simulink model "Final_openloop"  (R2024b)
settings: Solver=ode23s  StartTime=0.0  StopTime=150  RelTol=1e-3
(part 1 of 2)
settings Model: Creator=thomasmacbookpro  LastModifiedBy=thomasmacbookpro
settings OptimizationCC: ReuseModelBlockBuffer=off
settings RTWCC: GPUComputeCapability=3.5

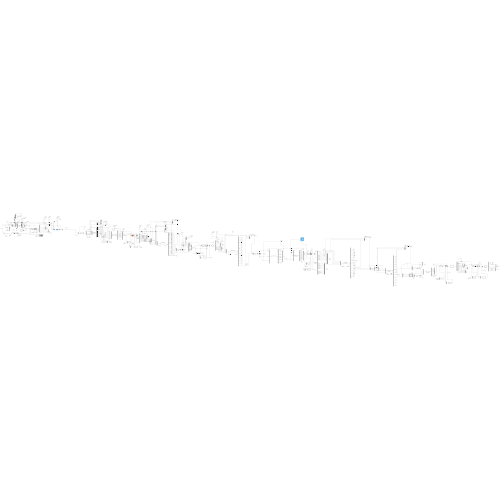
[thumbnail: Simulink's stored preview of the top-level diagram]
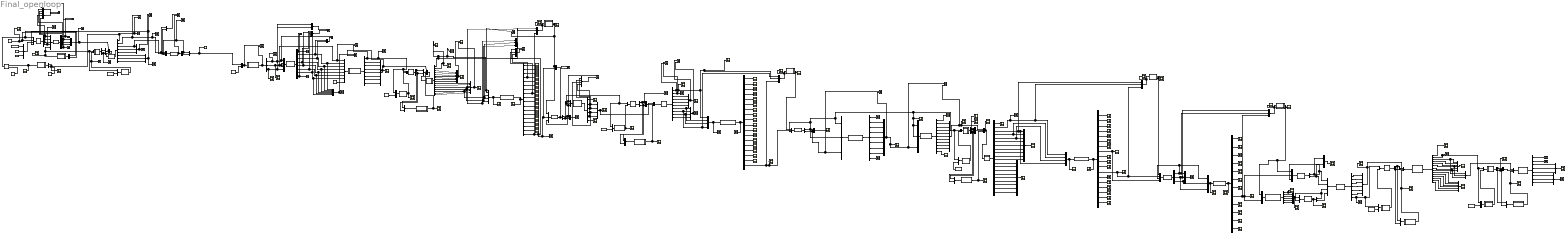
== system Final_openloop ==
  " Q, Recycle" : Scope
  AC-401:404 : S-Function  FunctionName=AC_Chromatography  Parameters=2  SFunctionDeploymentMode=off  EnableBusSupport=off
  AEX-201:204 : S-Function  FunctionName=AEX_Chromatography  Parameters=2  SFunctionDeploymentMode=off  EnableBusSupport=off
  AEX-301:304 : S-Function  FunctionName=AEX_Chromatography2  Parameters=2  SFunctionDeploymentMode=off  EnableBusSupport=off
  AEX:201:204 C : Scope  NumInputPorts=2
  AEX:201:204,Q IN/OUT1 : Scope  NumInputPorts=2
  "Area, UF-201" : Scope
  "Area, UF-301" : Scope
  "C, Glu, media [g/L]" : Constant  Value=18.1
  "C, N, media [g/L]" : Constant  Value=5.25
  "C, PE, 14" : Scope
  "C, PE, 22" : Scope
  "C, PE-1" : Scope
  "C, PE-2" : Scope
  "C, PE-3" : Scope
  "C, RE, 32" : Scope
  "C, RE, 4" : Scope
  "C, RE-1" : Scope
  "C, RE-2" : Scope
  "C, RE-3" : Scope
  "C, X, media [g/L]" : Constant  Value=0.22
  "C, alkaline lysis, out" : Scope
  "C, mRNA-LNP, PE, 48" : Scope
  "C, neutralization out" : Scope
  "C, output" : Scope
  "C,RE, 47" : Scope
  C,X : Scope
  CH3CO2K [M] : Constant  Value=3
  Constant : Constant  Value=2.72
  Constant1 : Constant  Value=0.8
  Delay block : VariableTransportDelay  VariableDelayType=Variable transport delay  MaximumDelay=10
  Delay time : Constant  Value=0.01
  Demux : Demux  Outputs=5
  Demux{1,5,9,32} (4 alike) : Demux  Outputs=8
  Demux10 : Demux  Outputs=18
  Demux{3..4,7,11,14,16,20,24..25,27,31} (11 alike) : Demux  Outputs=2
  Demux12 : Demux  Outputs=6
  Demux13 : Demux  Outputs=10
  Demux15 : Demux  Outputs=18
  Demux17 : Demux  Outputs=9
  Demux18 : Demux  Outputs=11
  Demux19 : Demux  Outputs=20
  Demux2 : Demux
  Demux21 : Demux  Outputs=18
  Demux22 : Demux  Outputs=12
  Demux23 : Demux  Outputs=3
  Demux26 : Demux  Outputs=7
  Demux28 : Demux  Outputs=14
  Demux29 : Demux  Outputs=6
  Demux6 : Demux  Outputs=16
  Demux8 : Demux  Outputs=3
  HIC-401:404 : S-Function  FunctionName=HIC_Chromatography  Parameters=2  SFunctionDeploymentMode=off  EnableBusSupport=off
  IVT : Scope
  "Input, AC-401:404" : Scope
  "Input, AEX-201:204" : Scope
  "Input, AEX-301:304" : Scope
  "Intput, HIC-401:404" : Scope
  M-101 : MATLAB Function  TreatAsAtomicUnit=on
  M-501 : S-Function  FunctionName=M_501  SFunctionDeploymentMode=off  EnableBusSupport=off
  MATLAB Function : MATLAB Function  TreatAsAtomicUnit=on
  MATLAB Function1 : MATLAB Function  TreatAsAtomicUnit=on
  MATLAB Function10 : MATLAB Function  TreatAsAtomicUnit=on
  MATLAB Function11 : MATLAB Function  TreatAsAtomicUnit=on
  MATLAB Function13 : MATLAB Function  TreatAsAtomicUnit=on
  MATLAB Function14 : MATLAB Function  TreatAsAtomicUnit=on
  MATLAB Function15 : MATLAB Function  TreatAsAtomicUnit=on
  MATLAB Function17 : MATLAB Function  TreatAsAtomicUnit=on
  MATLAB Function18 : MATLAB Function  TreatAsAtomicUnit=on
  MATLAB Function2 : MATLAB Function  TreatAsAtomicUnit=on
  MATLAB Function3 : MATLAB Function  TreatAsAtomicUnit=on
  MATLAB Function4 : MATLAB Function  TreatAsAtomicUnit=on
  MATLAB Function5 : MATLAB Function  TreatAsAtomicUnit=on
  MATLAB Function6 : MATLAB Function  TreatAsAtomicUnit=on
  MATLAB Function7 : MATLAB Function  TreatAsAtomicUnit=on
  MATLAB Function8 : MATLAB Function  TreatAsAtomicUnit=on
  MATLAB Function9 : MATLAB Function  TreatAsAtomicUnit=on
  MF-501 : MATLAB Function  TreatAsAtomicUnit=on
  MM-501 : MATLAB Function  TreatAsAtomicUnit=on
  Mux{,7,27,33..34,36..37,50,55,57,82,88} (12 alike) : Mux
  Mux{1,9..10,13..14,19..20,25..26,30,35,39..40,42,47,49,51,56,63,71..73,76,78,84..85,87,89..90} (29 alike) : Mux  Inputs=3
  Mux{3..6,8,11..12,15,21..22,28..29,31..32,38,44..45,52..54,59,61..62,65,67..70,74..75,77,79..81,83,86,91} (37 alike) : Mux  Inputs=2
  Mux{16..17,24,41} (4 alike) : Mux  Inputs=7
  Mux{18,58,60,64,66} (5 alike) : Mux  Inputs=6
  Mux2 : Mux  Inputs=5
  Mux23 : Mux  Inputs=8
  Mux43 : Mux  Inputs=9
  Mux46 : Mux  Inputs=9
  Mux48 : Mux  Inputs=9
  NF-501 : MATLAB Function  TreatAsAtomicUnit=on
  NaOH [M] : Constant  Value=0.42
  "Neutralization, IN/OUT2" : Scope  NumInputPorts=2
  Neutralization,flow IN/OUT1 : Scope  NumInputPorts=2
  "Output, AC-401:404" : Scope
  "Output, AEX-201:204" : Scope
  "Output, AEX-301:304" : Scope
  "Output, HIC-401:404" : Scope
  P : MATLAB Function  TreatAsAtomicUnit=on
  "Pressure MF-501, bar" : Constant  Value=1.4
  "Pressure NF-501, bar" : Constant  Value=8
  "Pressure UF-101, bar" : Constant  Value=1.85
  "Pressure UF-201, bar" : Constant  Value=1.85
  "Pressure UF-301, bar" : Constant  Value=1.85
  "Pressure UF-401, bar" : Constant  Value=1.85
  "Pressure, P" : Scope
  "Q, Out L/h" : MATLAB Function  TreatAsAtomicUnit=on
  "Q, PE" : Scope
  "Q, PE, 14" : Scope
  "Q, Pe-1" : Scope
  "Q, RE, 4" : Scope
  "Q, RE-1" : Scope
  R-101 : S-Function  FunctionName=CSTR  SFunctionDeploymentMode=off  EnableBusSupport=off
  "R-101, C out" : Scope
  "R-101, C:IN,OUT" : Scope  NumInputPorts=2
  "R-101, Level" : Scope
  "R-101, Volume" : Scope
  "R-101, Volume+height" : Scope  NumInputPorts=2
  R-201 : S-Function  FunctionName=Alkalinelysis  SFunctionDeploymentMode=off  EnableBusSupport=off
  "R-201, C,byproduct" : Scope  NumInputPorts=2
  "R-201, C,x" : Scope  NumInputPorts=2
  "R-201, Length " : Scope
  "R-201, Volume" : Scope
  "R-201, Volume+length" : Scope  NumInputPorts=2
  R-301 : S-Function  FunctionName=Linearization  SFunctionDeploymentMode=off  EnableBusSupport=off
  "R-301, C IN/OUT2" : Scope  NumInputPorts=2
  R-401 : S-Function  FunctionName=IVT  SFunctionDeploymentMode=off  EnableBusSupport=off
  "R-401, C IN/OUT1" : Scope  NumInputPorts=2
  R-402 : S-Function  FunctionName=Degradation_reactor  SFunctionDeploymentMode=off  EnableBusSupport=off
  "R-402, C IN/OUT2" : Scope  NumInputPorts=2
  "Resuspension, IN/OUT1" : Scope  NumInputPorts=2
  Rotational speed : Scope
  "Rotational speed, Rpm" : MATLAB Function  TreatAsAtomicUnit=on
  Scope{,1..108,111..112,126..127} (113 alike) : Scope
  T-101 : S-Function  FunctionName=T_101  SFunctionDeploymentMode=off  EnableBusSupport=off
  T-101 volume : Scope
  "T-101, out" : Scope
  T-205 : S-Function  FunctionName=T_205  SFunctionDeploymentMode=off  EnableBusSupport=off
  T-302 : S-Function  FunctionName=T_302  SFunctionDeploymentMode=off  EnableBusSupport=off
  T-402 : S-Function  FunctionName=T_402  SFunctionDeploymentMode=off  EnableBusSupport=off
  T-501 : S-Function  FunctionName=T_501  SFunctionDeploymentMode=off  EnableBusSupport=off
  "Tank-101, IN/OUT" : Scope  NumInputPorts=2
  "Tank-205, IN/OUT1" : Scope  NumInputPorts=2
  "Total flow, out" : Scope
  UF-101 : MATLAB Function  TreatAsAtomicUnit=on
  "UF-101, C, R/P" : Scope  NumInputPorts=2
  "UF-101, C, R/P1" : Scope  NumInputPorts=2
  "UF-101, Q, R/P" : Scope  NumInputPorts=2
  "UF-101, Q, R/P1" : Scope  NumInputPorts=2
  UF-201 : MATLAB Function  TreatAsAtomicUnit=on
  "UF-201, C, R/P2" : Scope  NumInputPorts=2
  "UF-201, Q, R/P2" : Scope  NumInputPorts=2
  UF-301 : MATLAB Function  TreatAsAtomicUnit=on
  UF-401 : MATLAB Function  TreatAsAtomicUnit=on
  VSP-101 : MATLAB Function  TreatAsAtomicUnit=on
  VSP-204 : MATLAB Function  TreatAsAtomicUnit=on
  "VSP-204, n" : Scope
  VSP-301 : MATLAB Function  TreatAsAtomicUnit=on
  "VSP-301, n" : Scope
  VSP-401 : MATLAB Function  TreatAsAtomicUnit=on
  VSP-503 : MATLAB Function  TreatAsAtomicUnit=on
  VSP-504 : MATLAB Function  TreatAsAtomicUnit=on
  wires:
  M-101/1(y) -> Demux2/1
  Mux/1 -> M-101/1(u)
  Demux2/2 -> Mux2/2, Mux71/2  "C, Glu"
  Demux2/1 -> Mux71/1, Mux2/1  "C, X"
  R-101/1 -> Demux/1
  Mux2/1 -> R-101/1
  Demux2/3 -> Mux71/3, Mux2/3  "C, N"
  Demux2/4 -> Scope126/1, Mux2/4  "Q, in"
  Mux14/1 -> Mux/3
  Demux/5 -> "R-101, Volume+height"/2, "R-101, Level"/1  "Level"
  Mux5/1 -> P/1(u)
  Constant/1 -> Scope105/1, Mux8/1, Mux/2  "Q, Media [L/h]"
  UF-101/1(y) -> Demux1/1
  Mux11/1 -> UF-101/1(u)
  Mux4/1 -> VSP-101/1(u)
  "Rotational speed, Rpm"/1(y) -> Rotational speed/1, Mux4/2  "Rotational speed, n"
  Mux1/1 -> "R-101, C out"/1, Mux11/1  "C, out"
  VSP-101/1(y) -> Demux3/1
  Demux3/1 -> Mux6/1  "Q"
  Mux6/1 -> Mux11/2
  Demux1/1 -> Mux5/1, "Q, PE"/1, "UF-101, Q, R/P"/2, "Q, Pe-1"/1  "Q,PE-1"
  Demux1/2 -> "UF-101, Q, R/P"/1, "Q, RE, 4"/1, Mux79/1, Mux9/1  "Q, RE. 4"
  Demux1/3 -> Mux13/1, Mux79/2, Mux9/2  "C, X, RE"
  Demux1/4 -> Mux13/2  "C, Glu, RE"
  Demux1/5 -> Mux13/3  "C, N, RE"
  Demux1/6 -> Mux10/1  "C, X, PE-1"
  Demux1/7 -> Mux10/2  "C, Glu, PE-1"
  Demux1/8 -> Mux10/3  "C, N, PE-1"
  Mux8/1 -> "Q, Out L/h"/1(u)
  "C, X, media [g/L]"/1 -> Mux14/1
  "C, N, media [g/L]"/1 -> Mux14/3
  "C, Glu, media [g/L]"/1 -> Mux14/2
  Mux9/1 -> T-101/1
  T-101/1 -> "Tank-101, IN/OUT"/2, Demux4/1
  Delay time/1 -> Delay block/2
  P/1(y) -> Delay block/1, " Q, Recycle"/1  "Q, Recycle [L/h]"
  Delay block/1 -> Mux8/2, Mux/1  "Q, Recycle [L/h]"
  R-201/1 -> Demux5/1
  Demux5/5 -> Mux18/4, Mux23/5, Mux82/2  "C, Denaturated plasmid"
  Demux5/3 -> Mux83/2, Mux18/2, Mux23/3  "C, Cell_disrupted"
  Demux5/1 -> "R-201, Volume+length"/1, "R-201, Volume"/1  "V"
  Demux5/6 -> Mux18/5, Mux23/6, Mux82/3  "C, Endotoxin"
  Demux5/4 -> Mux82/1, Mux18/3, Mux23/4  "C, pDNA"
  Demux5/2 -> Mux83/1, Mux18/1, Mux23/2  "C, Cell"
  Mux7/1 -> R-201/1
  Mux18/1 -> "Neutralization, IN/OUT2"/1, "C, alkaline lysis, out"/1
  Demux5/7 -> Mux82/4, Mux18/6, Mux23/7  "C, NaOH"
  Demux5/8 -> "R-201, Volume+length"/2, "R-201, Length "/1  "Length"
  Demux4/1 -> Mux21/1, T-101 volume/1, Mux9/3  "Q"
  MATLAB Function4/1(y) -> "Resuspension, IN/OUT1"/2, Demux8/1
  Demux4/2 -> Mux21/2  "C"
  Mux22/1 -> "Resuspension, IN/OUT1"/1, MATLAB Function4/1(u)
  Mux21/1 -> "T-101, out"/1, Mux22/1
  NaOH [M]/1 -> Mux22/2
  Demux8/1 -> C,X/1, Mux81/1, "R-201, C,x"/1, Mux7/1  "C, X"
  Demux8/3 -> Scope99/1, Mux81/2, Mux7/4  "C, NaOH"
  Demux8/2 -> Scope97/1, Neutralization,flow IN/OUT1/1, Mux23/1, Mux7/2, Mux7/3  "Q"
  Mux23/1 -> MATLAB Function5/1(u)
  MATLAB Function5/1(y) -> Demux9/1
  Demux9/2 -> Mux24/1  "C, Cell"
  Demux9/3 -> Mux24/2  "C, Cell_disrupted"
  Demux9/4 -> Mux24/3  "C, pDNA"
  Demux9/5 -> Mux24/4  "C, Denaturated plasmid"
  Demux9/6 -> Mux24/5  "C, Endotoxin"
  Demux9/7 -> Mux24/6  "C, NaOH"
  Demux6/8 -> Mux16/6  "C, NaOH, RE-1"
  Mux16/1 -> "UF-201, C, R/P2"/1, "C, RE-1"/1
  Demux6/4 -> Mux16/2  "C, Cell_disrupted, RE-1"
  MATLAB Function9/1(y) -> "VSP-204, n"/1, Mux12/2
  UF-201/1(y) -> Demux6/1
  Demux6/3 -> Mux16/1  "C, Cell, RE-1"
  Mux15/1 -> Mux19/2
  Demux6/7 -> Mux16/5  "C, Endotoxin, RE-1"
  Demux6/6 -> Mux16/4  "C, Denaturated plasmid, RE-1"
  Mux19/1 -> UF-201/1(u)
  VSP-204/1(y) -> Demux7/1
  Mux12/1 -> VSP-204/1(u)
  Demux6/5 -> Mux16/3  "C, pDNA, RE-1"
  Mux24/1 -> "C, neutralization out"/1, "Neutralization, IN/OUT2"/2, Mux19/1  "C, out"
  Mux17/1 -> "UF-201, C, R/P2"/2, "C, PE, 14"/1
  R-301/1 -> Demux12/1
  Demux12/2 -> Mux88/1, Mux34/1  "C, pDNA"
  CH3CO2K [M]/1 -> Mux23/8
  Demux9/8 -> Mux24/7  "C, CH3CO2K"
  Demux6/9 -> Mux16/7  "C, CH3CO2K, RE-1"
  Demux6/10 -> Mux17/1  "C, Cell, PE"
  Demux6/11 -> Mux17/2  "C, Cell_disrupted, PE"
  Demux6/12 -> Mux20/1, Mux17/3, Mux85/1, Mux27/4  "C, pDNA, PE"
  Demux6/13 -> Mux85/3, Mux27/3, Mux17/4  "C, Denaturated plasmid, PE"
  Demux6/14 -> Mux27/2, Mux85/2, Mux17/5  "C, Endotoxin, PE"
  Demux6/15 -> Mux17/6  "C, NaOH, PE"
  Demux6/16 -> Mux17/7  "C, CH3CO2K, PE"
  Demux10/14 -> Scope19/1
  Demux10/16 -> Scope8/1
  Demux10/2 -> Scope29/1
  Demux10/3 -> Scope30/1
  AEX-201:204/1 -> "Output, AEX-201:204"/1, Demux10/1
  Demux10/10 -> Scope23/1
  Demux10/7 -> Scope26/1
  Demux10/1 -> Scope28/1
  Demux10/11 -> Scope22/1
  Demux10/6 -> Scope5/1
  Demux10/15 -> Scope18/1
  Demux10/12 -> Scope21/1
  Demux10/4 -> Mux84/3, Scope2/1  "C, Denaturated plasmid"
  Demux10/13 -> Scope20/1
  Demux10/8 -> Mux84/2, Scope25/1  "C, Endotoxins"
  Demux10/9 -> Scope24/1
  Demux10/5 -> Scope13/1
  Demux10/17 -> Scope7/1
  Mux27/1 -> "Input, AEX-201:204"/1, AEX-201:204/1
  Mux30/1 -> T-205/1
  Demux11/1 -> Mux30/3, Mux31/1, Mux28/1, Mux26/2, Mux26/3, Mux29/1  "Q"
  Demux12/3 -> Mux88/2, Mux34/2  "C, linpDNA"
  Demux12/4 -> Mux88/3, Mux34/3  "C, Impurities"
  Demux11/2 -> Mux29/2, "R-301, C IN/OUT2"/1, Mux26/1  "C, pDNA"
  UF-301/1(y) -> Demux13/1
  Demux14/1 -> Mux67/1, Scope44/1, Mux32/1  "Q"
  Mux35/1 -> UF-301/1(u)
  Mux32/1 -> Mux35/2
  Demux14/2 -> Mux32/2, Mux67/2  "P"
  Demux13/2 -> "UF-101, Q, R/P1"/1, Scope34/1  "Q, RE-2"
  Mux31/1 -> VSP-301/1(u)
  Mux33/1 -> "UF-101, C, R/P1"/1, "C, RE-2"/1
  VSP-301/1(y) -> Demux14/1
  Demux12/5 -> Mux88/4, Mux34/4  "C, EcoRI enzyme"
  Demux13/3 -> Mux33/1  "C, pDNA, RE-2"
  Demux13/4 -> Mux33/2  "C, linpDNA, RE-2"
  Demux13/5 -> Mux33/3  "C, Impurities, RE-2"
  Demux13/6 -> Mux33/4  "C, EcoRI enzyme, RE-2"
  Demux13/9 -> Mux36/3, Mux37/3  "C, Impurities, PE"
  Demux13/10 -> Mux36/4  "C, ECoRI Enzyme, PE"
  Mux36/1 -> "UF-101, C, R/P1"/2, "C, PE, 22"/1
  Demux15/3 -> Scope47/1
  Demux15/1 -> Scope45/1
  Demux15/10 -> Scope41/1
  Demux15/4 -> Scope38/1  "C, Impurities"
  AEX-301:304/1 -> "Output, AEX-301:304"/1, Demux15/1
  Demux15/12 -> Scope52/1
  Mux37/1 -> AEX-301:304/1, "Input, AEX-301:304"/1
  Demux15/16 -> Scope50/1
  Demux15/9 -> Scope42/1
  Demux15/8 -> Scope53/1  "C, pDNA"
  Demux15/6 -> Scope48/1
  Demux15/14 -> Scope37/1
  Demux15/11 -> Scope40/1
  Demux15/2 -> Scope46/1
  Demux15/7 -> Scope43/1
  Demux15/5 -> Scope35/1
  Demux15/15 -> Scope36/1
  Demux15/17 -> Scope49/1
  Demux15/13 -> Scope39/1
  Mux39/1 -> T-302/1
  T-302/1 -> Demux16/1
  Demux17/5 -> Mux41/4  "C, linpDNA"
  Demux17/3 -> Mux41/2  "C, Impurities"
  Demux17/6 -> Mux41/5  "C, Cleancap"
  Demux16/1 -> Mux39/3, Mux54/1, Mux44/1, Scope17/1, Mux42/2, Mux42/1, Mux40/1, Mux40/2, Mux38/1  "Q"
  Demux16/2 -> "R-401, C IN/OUT1"/1, Mux40/3, Mux38/2  "C, linpDNA"
  R-401/1 -> Demux17/1
  Demux17/1 -> Scope55/1  "Volume"
  Demux17/2 -> Mux41/1  "C, mRNA"
  Mux40/1 -> R-401/1
  Demux17/4 -> Mux41/3  "C, T7 Enzyme"
  Demux17/8 -> Mux41/7  "C, Nucleotides"
  R-402/1 -> Demux18/1
  Demux18/2 -> Mux43/1  "C, mRNA"
  Demux18/3 -> Mux43/2  "C, Impurities"
  Demux18/4 -> Mux43/3  "C, T7 Enzyme"
  Demux18/5 -> Mux43/4  "C, linpDNA"
  Demux18/6 -> Mux43/5  "C, Cleancap"
  Demux18/8 -> Mux43/7  "C, Nucleotides"
  Demux18/9 -> Mux43/8  "C, Degraded products"
  Mux44/1 -> VSP-401/1(u)
  VSP-401/1(y) -> Demux20/1
  Mux45/1 -> Mux47/2
  UF-401/1(y) -> Demux19/1
  Demux19/4 -> Mux50/2, Mux46/2  "C, Impurities, RE"
  Demux19/5 -> Mux50/3, Mux46/3  "C, T7 Enzyme, RE"
  Demux19/6 -> Mux46/4  "C, linpDNA, RE"
  Demux19/7 -> Mux46/5  "C, CleanCap, RE"
  Demux19/9 -> Mux46/7  "C, Nucleotides, RE"
  Demux19/10 -> Mux46/8  "C, Degraded products, RE"
  Demux18/10 -> Mux43/9  "C, DNase I"
  Demux12/6 -> Scope63/1  "Level"
  Mux26/1 -> R-301/1
  Mux29/1 -> Scope6/1
  Mux34/1 -> "C, output"/1, Mux35/1
  Demux12/1 -> Scope12/1  "Volume"
  Mux46/1 -> "C, RE, 32"/1
  Mux48/1 -> "C, PE-2"/1
  Demux19/1 -> Scope60/1  "Q, PE-2"
  Mux42/1 -> R-402/1
  Demux18/11 -> Scope84/1  "Level"
  Demux23/3 -> Mux51/2, Mux49/3  "C, Impurities"
  Demux21/15 -> Scope66/1
  Demux21/1 -> Scope75/1
  Demux21/3 -> Scope77/1
  Demux21/10 -> Scope71/1
  Demux21/2 -> Scope76/1
  Demux21/6 -> Scope78/1
  Demux21/11 -> Scope70/1
  Demux21/17 -> Scope79/1
  Demux21/8 -> Mux55/4, Scope82/1  "C, impurities"
  Demux21/5 -> Scope58/1
  AC-401:404/1 -> "Output, AC-401:404"/1, Demux21/1
  Demux21/14 -> Scope67/1
  Demux21/16 -> Scope80/1
  Demux21/4 -> Scope68/1  "C, T7 enzyme"
  Demux21/9 -> Scope72/1
  Demux21/7 -> Scope73/1
  Demux21/13 -> Scope69/1
  Demux22/3 -> Scope87/1
  Demux22/10 -> Scope92/1
  Demux22/4 -> Scope101/1
  Demux22/6 -> Scope90/1  "C, Impurities"
  HIC-401:404/1 -> Demux22/1, "Output, HIC-401:404"/1
  Demux22/9 -> Scope93/1
  Demux22/7 -> Scope88/1
  Demux22/11 -> Scope91/1
  Mux51/1 -> "Intput, HIC-401:404"/1, HIC-401:404/1
  Mux50/1 -> AC-401:404/1, "Input, AC-401:404"/1
  Mux28/1 -> MATLAB Function8/1(u)
  "Pressure UF-301, bar"/1 -> Mux28/2
  MATLAB Function8/1(y) -> "VSP-301, n"/1, Mux31/2
  Mux52/1 -> MATLAB Function9/1(u)
  Demux9/1 -> Neutralization,flow IN/OUT1/2, Mux12/1, Mux52/1, "Total flow, out"/1  "Q, out"
  "Pressure UF-201, bar"/1 -> Mux52/2
  Mux53/1 -> "Rotational speed, Rpm"/1(u)
  "Q, Out L/h"/1(y) -> Scope106/1, Mux4/1, Mux53/1, Mux2/5  "Q1, out"
  "Pressure UF-101, bar"/1 -> Mux53/2
  Mux54/1 -> MATLAB Function11/1(u)
  Demux18/1 -> Scope65/1  "Volume"
  "Pressure UF-401, bar"/1 -> Mux54/2
  MATLAB Function11/1(y) -> Mux44/2
  Demux17/7 -> Mux41/6  "C, MgAcetate"
  Demux17/9 -> Scope56/1  "Level"
  Demux18/7 -> Mux43/6  "C, MgAcetate"
  Demux19/8 -> Mux46/6  "C, MgAcetate, RE"
  Demux19/11 -> Mux46/9  "C, DNase I ,RE"
  Demux19/12 -> Mux48/1  "C, mRNA, PE-2"
  Demux19/13 -> Mux48/2  "C, Impurities, PE-2"
  Demux19/14 -> Mux48/3  "C, T7 enzyme, PE-2"
  Demux19/15 -> Mux48/4  "C, linpDNA, PE-2"
  Demux19/16 -> Mux48/5  "C, CleanCap, PE-2"
  Demux19/17 -> Mux48/6  "C, MgAcetate, PE-2"
  Demux19/18 -> Mux48/7  "C, Nucleotides, PE-2"
  Demux19/19 -> Mux48/8  "C, Degraded products, PE-2"
  Demux19/20 -> Mux48/9  "C, DNase I, PE-2"
  Mux55/1 -> T-402/1
  T-402/1 -> Demux23/1
  Mux62/1 -> Mux63/2
  Demux25/2 -> Mux57/4  "C, solution"
  Mux64/1 -> Mux63/1, Scope51/1
  Demux28/3 -> Mux78/1, Mux58/1  "C, mRNA-LNP, RE"
  Mux61/1 -> VSP-503/1(u)
  Mux63/1 -> NF-501/1(u)
  T-501/1 -> Demux24/1
  Demux24/1 -> Mux91/1, Mux57/1, Mux56/3  "Q, TankF"
  MM-501/1(y) -> Demux26/1
  Mux57/1 -> MM-501/1(u)
  Mux58/1 -> "C,RE, 47"/1
  Demux28/4 -> Mux58/2  "C, LNP, RE"
  Demux25/1 -> Mux57/3, Mux70/2  "Q, TankG"
  Demux28/2 -> Scope112/1, Mux77/1, Mux74/1  "Q, RE-3"
  Demux24/2 -> Mux91/2, Mux57/2  "C, mRNA"
  Mux56/1 -> T-501/1
  VSP-503/1(y) -> Demux27/1
  M-501/1 -> Scope104/1, Demux25/1
  Demux28/6 -> Mux78/2, Mux58/4  "C, Sucroce, RE"
  Demux28/5 -> Mux58/3  "C, Ethanol, RE"
  NF-501/1(y) -> Demux28/1
  Mux65/1 -> MATLAB Function13/1(u)
  "Pressure NF-501, bar"/1 -> Mux65/2
  MATLAB Function13/1(y) -> Mux61/2
  Demux28/1 -> Scope111/1  "Q, PE, 47"
  Mux60/1 -> "C, PE-3"/1
  Mux72/1 -> "C, RE-3"/1
  VSP-504/1(y) -> Demux31/1
  Mux73/1 -> "C, mRNA-LNP, PE, 48"/1
  Demux32/2 -> Scope3/1  "Q, RE-3"
  Demux31/2 -> Scope98/1, Mux80/2, Mux75/2  "P"
  MF-501/1(y) -> Demux32/1
  Demux32/1 -> Scope127/1  "Q, PE, 48"
  Demux32/3 -> Mux72/1  "C, mRNA-LNP, RE-3"
  Mux74/1 -> VSP-504/1(u)
  Mux75/1 -> Mux76/2
  Mux76/1 -> MF-501/1(u)
  Mux77/1 -> MATLAB Function17/1(u)
  MATLAB Function17/1(y) -> Mux74/2
  "Pressure MF-501, bar"/1 -> Mux77/2
  Demux32/4 -> Mux72/2  "C, Sucrose, RE-3"
  Mux78/1 -> Mux76/1
  MATLAB Function1/1(y) -> Demux29/1
  Mux3/1 -> MATLAB Function1/1(u)
  Mux70/1 -> M-501/1
  Demux29/1 -> Scope16/1, Mux66/1  "Q, total"
  Demux29/2 -> Mux66/2  "C, LNP"
  Demux29/3 -> Mux66/3  "C, Ethanol"
  Demux29/4 -> Mux66/4  "C, sucrose"
  Demux29/5 -> Mux66/5  "C, Impurity 1"
  Mux66/1 -> Scope57/1, Mux70/1
  Demux26/2 -> Mux64/2  "C, LNP"
  Demux26/3 -> Mux64/3  "C, Ethanol"
  Demux26/4 -> Mux64/4  "C, Sucrose 1"
  MATLAB Function3/1(y) -> "Area, UF-301"/1, Mux35/3
  Mux67/1 -> MATLAB Function3/1(u)
  Mux69/1 -> MATLAB Function6/1(u)
  MATLAB Function6/1(y) -> "Area, UF-201"/1, Mux19/3
  Demux7/1 -> Mux69/1, Mux15/1  "Q"
  Demux7/2 -> Mux15/2, Mux69/2  "P"
  Mux68/1 -> MATLAB Function14/1(u)
  MATLAB Function14/1(y) -> Mux47/3, Scope102/1
  Demux20/1 -> Scope31/1, Mux68/1, Mux45/1  "Q"
  Demux20/2 -> Scope32/1, Mux68/2, Mux45/2  "P"
  Mux59/1 -> MATLAB Function15/1(u)
  MATLAB Function15/1(y) -> Scope107/1, Mux63/3
  Demux27/1 -> Mux59/1, Mux62/1  "Q"
  Demux27/2 -> Mux59/2, Mux62/2  "P"
  MATLAB Function18/1(y) -> Scope108/1, Mux76/3
  Demux31/1 -> Mux80/1, Mux75/1  "Q"
  Mux80/1 -> MATLAB Function18/1(u)
  Demux22/5 -> Scope100/1
  Demux22/2 -> Scope85/1
  Demux22/1 -> Scope89/1
  Demux29/6 -> Mux66/6  "C, Impurity 2"
  Demux26/5 -> Mux64/5  "C, Impurity 1"
  Demux28/7 -> Mux58/5  "C, Impurity 1, RE"
  Demux32/5 -> Mux72/3  "C, Impurity 2, RE-3"
  Demux32/6 -> Mux73/1  "C, mRNA-LNP, PE"
  Demux32/7 -> Mux73/2  "C, Sucrose, PE"
  Demux32/8 -> Mux73/3  "C, Impurity 2, PE"
  Demux/4 -> Mux25/3, Mux1/3  "C, N"
  Demux/3 -> Mux1/2, Mux25/2  "C, Glu"
  Demux/2 -> Mux25/1, Mux1/1  "C, X"
  Mux47/1 -> Scope27/1, UF-401/1(u)
  Mux38/1 -> Scope54/1
  Demux26/1 -> Mux64/1  "C, mRNA-LNP"
  Demux/1 -> "R-101, Volume+height"/1, "R-101, Volume"/1  "V"
  Mux49/1 -> Scope4/1
  Mux13/1 -> "UF-101, C, R/P"/1, "C, RE, 4"/1
  Demux3/2 -> "Pressure, P"/1, Mux6/2  "P"
  Mux71/1 -> "R-101, C:IN,OUT"/1
  Mux25/1 -> "R-101, C:IN,OUT"/2
  Mux10/1 -> "UF-101, C, R/P"/2, Mux/4, "C, PE-1"/1
  Mux79/1 -> "Tank-101, IN/OUT"/1
  Mux81/1 -> "R-201, C,byproduct"/1
  Mux82/1 -> "R-201, C,byproduct"/2
  Mux83/1 -> "R-201, C,x"/2
  Demux6/2 -> "UF-201, Q, R/P2"/1, "Q, RE-1"/1  "Q, RE. 4"
  Mux84/1 -> AEX:201:204 C/2
  Mux85/1 -> AEX:201:204 C/1
  T-205/1 -> "Tank-205, IN/OUT1"/2, Demux11/1
  Mux86/1 -> "Tank-205, IN/OUT1"/1
  Demux6/1 -> Mux20/2, "UF-201, Q, R/P2"/2, AEX:201:204,Q IN/OUT1/1, Mux27/1, "Q, PE, 14"/1  "Q, RE. 4"
  Demux10/18 -> Mux86/2, Mux30/2, Scope/1, Mux84/1, Mux20/3  "C, pDNA,  RE"
  Mux88/1 -> "R-301, C IN/OUT2"/2
  Mux41/1 -> "R-401, C IN/OUT1"/2, IVT/1, "R-402, C IN/OUT2"/1, Mux42/3
  Mux43/1 -> "R-402, C IN/OUT2"/2, Scope9/1, Mux47/1
  Demux21/18 -> Scope14/1  "C, mRNA"
  Demux22/12 -> Scope15/1  "C, mRNA"
  Mux20/1 -> Scope62/1, MATLAB Function/1(u)
  Demux13/8 -> Mux36/2, Mux87/1, Mux37/4  "C, linpDNA, PE"
  Demux13/1 -> "UF-101, Q, R/P1"/2, Scope33/1, Mux87/2, Scope11/1, Mux37/1  "Q, RE. 4"
  Demux13/7 -> Mux36/1, Mux37/2  "C, pDNA, PE"
  Mux87/1 -> Scope74/1, MATLAB Function2/1(u)
  Demux15/18 -> Mux87/3, Scope10/1, Mux39/2  "C, pDNA,  RE"
  MATLAB Function2/1(y) -> Mux39/1, Scope64/1
  Demux19/3 -> Mux89/1, Mux50/4, Mux46/1  "C, mRNA, PE"
  Demux19/2 -> Scope1/1, Mux89/2, Mux50/1  "Q, RE. 4"
  MATLAB Function7/1(y) -> Mux55/1, Scope83/1
  Mux89/1 -> Scope86/1, MATLAB Function7/1(u)
  Demux21/12 -> Mux89/3, Mux55/2, Scope81/1  "C, mRNA,  RE"
  Mux90/1 -> Scope95/1, MATLAB Function10/1(u)
  Demux23/1 -> Mux90/2, Mux49/1, Mux55/3, Mux51/1  "Q, RE. 4"
  Demux23/2 -> Mux51/3, Mux90/1, Mux49/2  "C, mRNA, PE"
  Demux22/8 -> Mux90/3, Mux56/2, Mux3/2, Scope103/1  "C, mRNA,  RE"
  MATLAB Function10/1(y) -> Mux3/1, Mux56/1, Scope94/1
  MATLAB Function/1(y) -> Mux86/1, Mux30/1, AEX:201:204,Q IN/OUT1/2, Scope61/1
  Mux91/1 -> Scope59/1
  Demux26/6 -> Mux64/6  "C, Impurity 2"
  Demux26/7 -> Scope96/1, Mux65/1, Mux61/1  "Q, total"
  Demux28/8 -> Mux78/3, Mux58/6  "C,imurity 2 PE-3"
  Demux28/9 -> Mux60/1  "C, mRNA-LNP, PE-3"
  Demux28/10 -> Mux60/2  "C, LNP, PE-3"
  Demux28/11 -> Mux60/3  "C, Ethanol, PE-3"
  Demux28/12 -> Mux60/4  "C, Sucrose, PE-3"
  Demux28/13 -> Mux60/5  "C, Impurity 1, PE-3"
  Demux28/14 -> Mux60/6  "C, Impurity 2, PE-3"
  Constant1/1 -> Mux5/2  "Q, Media [L/h]"

== matlab function Final_openloop/M-101 ==
  data: y output; u input
function y  = MX(u) 

% inputs
Q_R = u(1);     % Recycling stream
Q_M = u(2);     % Fresh media stream
C_X_M = u(3);   % Fresh biomass concentration
C_GLU_M = u(4); % Fresh glucose concentration
C_N_M = u(5);   % Fresh nitrogen concentration
C_X_S = u(6);   % Recycle biomass concentration
C_GLU_S = u(7); % Recycle glucose concentration
C_N_S = u(8);   % Recycle nitrogen concentration


% output
y=zeros(4,1);
y(1) = (C_X_S*Q_R+C_X_M*Q_M)/(Q_M+Q_R);         %C_X_F
y(2) = (C_GLU_M*Q_M+C_GLU_S*Q_R)/(Q_M+Q_R);     %C_GLU_F
y(3) = (C_N_M*Q_M+C_N_S*Q_R)/(Q_M+Q_R);         %C_N_F
y(4) = (Q_M+Q_R);                               % Q_F

== matlab function Final_openloop/MATLAB Function8 ==
  data: u input; y output
function y = Rotationalspeed_n(u)

% inputs
Q=u(1);
P=u(2);


n=1.057500000*Q + 3.286399171*10^(-9)*sqrt(5.060362715*10^20*Q^2 + 6.085688000*10^22*P);

y=zeros(1,1);
y(1) = (n); %n

== matlab function Final_openloop/MATLAB Function9 ==
  data: u input; y output
function y = n(u)

% inputs
Q=u(1);
P=u(2);


n=1.057500000*Q + 3.286399171*10^(-9)*sqrt(5.060362715*10^20*Q^2 + 6.085688000*10^22*P);

y=zeros(1,1);
y(1) = (n); %n

== matlab function Final_openloop/Rotational speed, Rpm ==
  data: u input; y output
function y = n(u)

% inputs
Q=u(1);
P=u(2);


n=1.057500000*Q + 3.286399171*10^(-9)*sqrt(5.060362715*10^20*Q^2 + 6.085688000*10^22*P);

y=zeros(1,1);
y(1) = (n); % n

== matlab function Final_openloop/MATLAB Function11 ==
  data: u input; y output
function y = n(u)

% inputs
Q=u(1);
P=u(2);


n=1.057500000*Q + 3.286399171*10^(-9)*sqrt(5.060362715*10^20*Q^2 + 6.085688000*10^22*P);

y=zeros(1,1);
y(1) = (n); %n

== matlab function Final_openloop/MM-501 ==
  data: y output; u input
function y  = MX(u)

% Inputs: [Q_F, C_mRNA_F, Q_G, C_LNP_G, C_ethanol_G, C_imp1_G, C_imp2_G, C_imp3_G, encapsulation_efficiency]

% Inputs
Q_F = u(1);                                      % Flow rate from Tank F (mRNA solution)
C_mRNA_F = u(2);                                 % mRNA concentration
Q_G = u(3);                                      % Flow rate from Tank G (LNP solution)
C_LNP_G = u(4);                                  % LNP concentration (Tank G)
C_ethanol_G = u(5);                              % Ethanol concentration
C_sucrose_G = u(6);                              % Sucrose concentration
C_imp1_G = u(7);                                 % Impurity 1 concentration 
C_imp2_G = u(8);                                 % Impurity 2 concentration

y = zeros(7, 1);

y(1) = (C_mRNA_F * Q_F)/(Q_F + Q_G);       % Encapsulated mRNA-LNP (assumed 100% encapsulated)
y(2) = (C_LNP_G * Q_F)/(Q_F + Q_G);       % Encapsulated LNP (assumed 100% encapsulated)
y(3) = (C_ethanol_G* Q_G) / (Q_F + Q_G);         % C_ethanol
y(4) = (C_sucrose_G* Q_G) / (Q_F + Q_G);         % C_ethanol
y(5) = (C_imp1_G * Q_G) / (Q_F + Q_G);           % C_Impurity 1
y(6) = (C_imp2_G * Q_G) / (Q_F + Q_G);           % C_Impurity 2
y(7) = (Q_F + Q_G);                                % Total flow rate

end

== matlab function Final_openloop/NF-501 ==
  data: u input; y output
function y = NF(u)
%% parameters for nanofiltration 
% a DOW NF90 nanofiltration membrane has been chosen. This type of membrane
% has been used in pharmaceutical applications for API filtrations (title
% reference: Removal of antibiotics from a model wastewater by RO/NF membranes)
%A=0.398443840087261; %membrane surface area [m^2] 
%% parameters for nanofiltration 
%A=0.3984033;
Jw=57.90; %permeate flowrate at 8 bar pressure [l/m^2/h]
Res=Jw/8; %[l/m^2/h/bar]function y  = NN(u)


%input
C_mRNALNP_4=u(1);
C_LNP_4=u(2);
C_Ethanol_4=u(3);
C_Sucrose_4=u(4);
C_IMP1_4=u(5);
C_IMP2_4=u(6);
Q_IN=u(7);
P=u(8);
A=u(9);

tlim=1;
dim=14;
y=zeros(dim,1);


%% Rejection coefficients for different species
Rej=[0.00002*P^4 - 0.0018*P^3 + 0.0145*P^2 + 0.0849*P + 0.22248; 0.01; 0.01; 0.00002*P^4 - 0.0018*P^3 + 0.0145*P^2 + 0.0849*P + 0.22248; 0.01; 0.99];


%% Output calculations

     y(1)=A*Res*P;%permeate volumetric flowrate [l/h];(ref: Continuous purification of
    %active pharmaceutical ingredients using multistage organic solvent nanofiltration membrane cascade)
    y(2)=Q_IN-y(1); %balance on centrifugation+filtration
    

%% Species balances for retentate stream (calculated based on inflow and rejection)
    y(3)=(Q_IN*C_mRNALNP_4)/(y(2)+y(1)*(1-Rej(1)));         % mRNA-LNP concentration in retentate stream
    y(4)=(Q_IN*C_LNP_4)/(y(2)+y(1)*(1-Rej(2)));         % LNP concentration in retentate stream
    y(5)=(Q_IN*C_Ethanol_4)/(y(2)+y(1)*(1-Rej(3)));         % Ethanol concentration in retentate stream
    y(6)=(Q_IN*C_Sucrose_4)/(y(2)+y(1)*(1-Rej(4)));         % Sucrose concentration in retentate stream
    y(7)=(Q_IN*C_IMP1_4)/(y(2)+y(1)*(1-Rej(5)));            % Impurity 1 concentration in retentate stream
    y(8)=(Q_IN*C_IMP2_4)/(y(2)+y(1)*(1-Rej(6)));            % Impurity 2 concentration in retentate stream
   
 %% Species concentrations in permeate stream (calculated based on rejection)
    y(9)=y(3)*(1-Rej(1));                                   % mRNA-LNP concentration in permeate stream
    y(10)=y(4)*(1-Rej(2));                                   % LNP concentration in permeate stream
    y(11)=y(5)*(1-Rej(3));                                   % Ethanol concentration in permeate stream
    y(12)=y(6)*(1-Rej(4));                                  % Sucrose concentration in permeate stream
    y(13)=y(7)*(1-Rej(5));                                  % Impurity 1 concentration in permeate stream
    y(14)=y(8)*(1-Rej(6));                                  % Impurity 2 concentration in permeate stream
  

end

== matlab function Final_openloop/VSP-503 ==
  data: u input size=2; y output size=2
function y  = Pump(u)

%input
Q_C=u(1);
n=u(2);


y=zeros(2,1);

% output

y(1)=Q_C;
y(2)=((-0.085*Q_C^2 - 0.0000329*Q_C*n + 0.0000155555555555556*n^2)*(997*9.81))/10^5;


end

== matlab function Final_openloop/MATLAB Function13 ==
  data: u input; y output
function y = n(u)

% inputs
Q=u(1);
P=u(2);


n=1.057500000*Q + 3.286399171*10^(-9)*sqrt(5.060362715*10^20*Q^2 + 6.085688000*10^22*P);

y=zeros(1,1);
y(1) = (n); %n

== matlab function Final_openloop/MATLAB Function1 ==
  data: u input; y output
function y = Formulation_medium(u)
    % Inputs
    Q = u(1);                                   % Total flow rate (L/h)
    C_mRNA = u(2);                              % Concentration of mRNA (g/L)

    % Distribution of flow rates
    Q_Ethanol = Q/3;                            % Ethanol flow (1/3 of total flow)
    Q_LNP = Q / 3;                              % LNP flow (1/3 of total flow)
    Q_Sucrose = Q*10;                            % LNP flow (1/3 of total flow)

    % Concentrations
    C_LNP = C_mRNA / 0.029;                     % LNP concentration (g/g)
    C_Sucrose = Q_Sucrose *0.1;                   % Sucrose concentration
    C_Impurities_1 = Q_Ethanol * 0.05;          % Impurity 1: 5% of ethanol flow
    C_Impurities_2 = Q_Ethanol * 0.05;          % Impurity 2: 5% of ethanol flow

    % Outputs
    y = zeros(1, 6); % Output vector
    y(1) = (Q_Ethanol + Q_LNP + Q_Sucrose);       % Total flow rate (ethanol + LNP)
    y(2) = (C_LNP * Q_LNP) / y(1);              % Weighted concentration of LNP
    y(3) = (Q_Ethanol) / y(1);        % Weighted Ethanol concentration
    y(4) = (C_Sucrose*Q_Sucrose) / y(1);        % Weighted Sucrose concentration
    y(5) = (C_Impurities_1 * Q_Ethanol) / y(1); % Weighted concentration of Impurity 1
    y(6) = (C_Impurities_2 * Q_Ethanol) / y(1); % Weighted concentration of Impurity 2
end

== matlab function Final_openloop/MATLAB Function3 ==
  data: u input; y output
function y = Membrane_area(u)
    % Inputs
    Q_IN = u(1);  % Total flow rate (L/h)
    P = u(2);     % Pressure (kPa)

    % Parameters for nanofiltration
    P_0 = 0.49;        % Reference pressure (kPa)
    alpha_0 = 10.2 * 10^12; % Reference alpha (kPa*s)^-1
    n = 0.5;            % Exponent for alpha
    eta_perm = 1.0 * 10^-8;  % Viscosity (kPa*s)
    m_x_c = 7.7 * 10^-3;    % Membrane permeability coefficient (kg)
    R_m = 1.26 * 10^12;     % Membrane resistance (1/m)

    % Calculate alpha based on the pressure
    alpha = alpha_0 * (P / P_0)^n;

    % Desired permeate flow is 40% of Q_IN
    desired_permeate_flow = 0.8 * Q_IN;

    % Initial guess for membrane area A (in m^2)
    A_min = 1e-6;   % Min value for area (to avoid division by zero)
    A_max = 10;     % Max value for area (arbitrary large number)
    tolerance = 1e-6;  % Tolerance for solution accuracy
    max_iter = 100;  % Maximum number of iterations

    % Bisection method to find A
    for iter = 1:max_iter
        A_mid = (A_min + A_max) / 2;
        
        % Calculate R_C based on A_mid
        R_C_mid = alpha * m_x_c / A_mid;

        % Calculate permeate flow based on A_mid
        permeate_flow = (P / (eta_perm * (R_m + R_C_mid))) * A_mid * 1000 * 3600;

        % Check if the calculated permeate flow is close to the desired value
        if abs(permeate_flow - desired_permeate_flow) < tolerance
            break;
        elseif permeate_flow > desired_permeate_flow
            A_max = A_mid;  % Search in the lower half
        else
            A_min = A_mid;  % Search in the upper half
        end
    end

    % The solution found for A is stored in A_mid
    A_value = A_mid;

    % Output the membrane area (in m^2)
    y = A_value;  % Membrane area (m^2)
end

== matlab function Final_openloop/P ==
  data: u input; y output
function y = Purge(u)

% inputs
Q_R=u(1);
Q_P=u(2);


y=zeros(1,1);
y(1) = Q_R*Q_P; % recycle stream

== matlab function Final_openloop/MATLAB Function6 ==
  data: u input; y output
function y = Membrane_area(u)
    % Inputs
    Q_IN = u(1);                    % Total flow rate (L/h)
    P = u(2);                       % Pressure (kPa)

    % Parameters for nanofiltration
    P_0 = 0.49;                     % Reference pressure (kPa)
    alpha_0 = 10.2 * 10^12;         % Reference alpha (kPa*s)^-1
    n = 0.5;                        % Exponent for alpha
    eta_perm = 1.0 * 10^-8;         % Viscosity (kPa*s)
    m_x_c = 7.7 * 10^-3;            % Membrane permeability coefficient (kg)
    R_m = 1.26 * 10^12;             % Membrane resistance (1/m)

    % Calculate alpha based on the pressure
    alpha = alpha_0 * (P / P_0)^n;

    % Desired permeate flow is 80% of Q_IN
    desired_permeate_flow = 0.8 * Q_IN;

    % Initial guess for membrane area A (in m^2)
    A_min = 1e-6;                   % Min value for area (to avoid division by zero)
    A_max = 10;                     % Max value for area (arbitrary large number)
    tolerance = 1e-6;               % Tolerance for solution accuracy
    max_iter = 100;                 % Maximum number of iterations

    % Bisection method to find A
    for iter = 1:max_iter
        A_mid = (A_min + A_max) / 2;
        
        % Calculate R_C based on A_mid
        R_C_mid = alpha * m_x_c / A_mid;

        % Calculate permeate flow based on A_mid
        permeate_flow = (P / (eta_perm * (R_m + R_C_mid))) * A_mid * 1000 * 3600;

        % Check if the calculated permeate flow is close to the desired value
        if abs(permeate_flow - desired_permeate_flow) < tolerance
            break;
        elseif permeate_flow > desired_permeate_flow
            A_max = A_mid;          % Search in the lower half
        else
            A_min = A_mid;          % Search in the upper half
        end
    end

    % The solution found for A is stored in A_mid
    A_value = A_mid;

    % Output the membrane area (in m^2)
    y = A_value;                    % Membrane area (m^2)
end

== matlab function Final_openloop/MF-501 ==
  data: u input; y output
function y  = MF(u)

%input
C_mRNALNP_4=u(1);
C_sucrose_4=u(2);
C_IMP2_4=u(3);
Q_IN=u(4);
P=u(5);
A=u(6);

%% parameters for microfiltration 

%A=0.00045; %m^2
Jw=800;                 % Permeate flowrate at 1.4 bar pressure [l/m^2/h]
Res=Jw/P;               % [l/m^2/h/bar]function y  = NN(u)

tlim=1;                 % h
dim=8;
y=zeros(dim,1);


%% Rejection coefficients for different species
Rej=[0.01; 0.01; -0.048272*P^4-0.035917*P^3+0.087656*P^2+0.49559*P+0.40839];

%% Output calculations

    y(1)=A*Res*P;       % permeate volumetric flowrate [l/h];(ref: Continuous purification of active pharmaceutical ingredients using multistage organic solvent nanofiltration membrane cascade)
    y(2)=Q_IN-y(1);     % balance on centrifugation+filtration
    
%% Species balances for retentate stream (calculated based on inflow and rejection)
    y(3)=(Q_IN*C_mRNALNP_4)/(y(2)+y(1)*(1-Rej(1)));         % mRNA-LNP in retentate stream
    y(4)=(Q_IN*C_sucrose_4)/(y(2)+y(1)*(1-Rej(2)));         % Sucrose in retentate stream
    y(5)=(Q_IN*C_IMP2_4)/(y(2)+y(1)*(1-Rej(3)));            % Impurity 2 in retentate stream
   
 %% Species concentrations in permeate stream (calculated based on rejection)
    y(6)=y(3)*(1-Rej(1));                                   % mRNA-LNP in permeate stream
    y(7)=y(4)*(1-Rej(2));                                   % Sucrose in permeate stream
    y(8)=y(5)*(1-Rej(3));                                   % Impurity 2 permeate
    
end

== matlab function Final_openloop/MATLAB Function17 ==
  data: u input; y output
function y = n(u)

% inputs
Q=u(1);
P=u(2);


n=1.057500000*Q + 3.286399171*10^(-9)*sqrt(5.060362715*10^20*Q^2 + 6.085688000*10^22*P);

y=zeros(1,1);
y(1) = (n); %n

== matlab function Final_openloop/VSP-504 ==
  data: u input size=2; y output size=2
function y  = Pump(u)

%input
Q_C=u(1);
n=u(2);


y=zeros(2,1);

% output

y(1)=Q_C;
y(2)=((-0.085*Q_C^2 - 0.0000329*Q_C*n + 0.0000155555555555556*n^2)*(997*9.81))/10^5;


end

== matlab function Final_openloop/MATLAB Function ==
  data: u input; y output
function y = Flow(u)
% Flow Function to calculate the required flow rate for a given concentration
% Inputs:
% u(1) - C1: Original concentration (g/L)
% u(2) - f1: Original flow rate (L/h)
% u(3) - C2: New concentration (g/L)
%
% Output:
% y - f2: Required flow rate (L/h) to achieve the same total mass flow T

% Input assignments
C1 = u(1);  % Original concentration (g/L)
f1 = u(2);  % Original flow rate (L/h)
C2 = u(3);  % New concentration (g/L)

% Calculate the required flow rate f2
y = (C1 * f1) / C2;  % New flow rate to maintain the same total mass flow

% Ensure the output is between 5 and 8
if y < 0.000001
    y = 0.000001;
elseif y > 8
    y = 8;
end

end

== matlab function Final_openloop/MATLAB Function14 ==
  data: u input; y output
function y = Membrane_area(u)
    % Inputs
    Q_IN = u(1);  % Total flow rate (L/h)
    P = u(2);     % Pressure (kPa)

    % Parameters for nanofiltration
    P_0 = 0.49;        % Reference pressure (kPa)
    alpha_0 = 10.2 * 10^12; % Reference alpha (kPa*s)^-1
    n = 0.5;            % Exponent for alpha
    eta_perm = 1.0 * 10^-8;  % Viscosity (kPa*s)
    m_x_c = 7.7 * 10^-3;    % Membrane permeability coefficient (kg)
    R_m = 1.26 * 10^12;     % Membrane resistance (1/m)

    % Calculate alpha based on the pressure
    alpha = alpha_0 * (P / P_0)^n;

    % Desired permeate flow is 80% of Q_IN
    desired_permeate_flow = 0.8 * Q_IN;

    % Initial guess for membrane area A (in m^2)
    A_min = 1e-6;   % Min value for area (to avoid division by zero)
    A_max = 10;     % Max value for area (arbitrary large number)
    tolerance = 1e-6;  % Tolerance for solution accuracy
    max_iter = 100;  % Maximum number of iterations

    % Bisection method to find A
    for iter = 1:max_iter
        A_mid = (A_min + A_max) / 2;
        
        % Calculate R_C based on A_mid
        R_C_mid = alpha * m_x_c / A_mid;

        % Calculate permeate flow based on A_mid
        permeate_flow = (P / (eta_perm * (R_m + R_C_mid))) * A_mid * 1000 * 3600;

        % Check if the calculated permeate flow is close to the desired value
        if abs(permeate_flow - desired_permeate_flow) < tolerance
            break;
        elseif permeate_flow > desired_permeate_flow
            A_max = A_mid;  % Search in the lower half
        else
            A_min = A_mid;  % Search in the upper half
        end
    end

    % The solution found for A is stored in A_mid
    A_value = A_mid;

    % Output the membrane area (in m^2)
    y = A_value;  % Membrane area (m^2)
end

== matlab function Final_openloop/MATLAB Function15 ==
  data: u input; y output
function y = membrane_area(u)
    % Inputs
    Q_IN = u(1);  % Total flow rate (L/h)
    P = u(2);     % Pressure (kPa)

    % Parameters
    Jw = 57.90;       % Permeate flow rate at 8 bar pressure [L/m^2/h]
    Res = Jw / 8;     % Permeability [L/m^2/h/bar]
    desired_permeate_flow = 0.8 * Q_IN; % Desired permeate flow [L/h]

    % Initial bounds for membrane area A (m^2)
    A_min =0.01;  % Minimum possible area
    A_max = 10;    % Arbitrary maximum area
    tolerance = 1e-6;  % Tolerance for convergence
    max_iter = 100;    % Maximum iterations for bisection method

    % Bisection method to find A
    for iter = 1:max_iter
        % Midpoint of current range for A
        A_mid = (A_min + A_max) / 2;

        % Calculate permeate flow using the updated equation
        permeate_flow = A_mid * Res * P; % [L/h]

        % Check convergence
        if abs(permeate_flow - desired_permeate_flow) < tolerance
            break;  % Converged to the solution
        elseif permeate_flow > desired_permeate_flow
            A_max = A_mid;  % Adjust upper bound
        else
            A_min = A_mid;  % Adjust lower bound
        end
    end

    % Output the membrane area
    y = A_mid;  % Membrane area (m^2)
end

== matlab function Final_openloop/MATLAB Function18 ==
  data: u input; y output
function y = Membrane_area(u)
    % Inputs
    Q_IN = u(1);  % Total flow rate (L/h)
    P = u(2);     % Pressure (kPa)

    % Parameters
    Jw=800; %permeate flowrate at 1.4 bar pressure [l/m^2/h]
    Res=Jw/P; %[l/m^2/h/bar]function y  = NN(u)
    desired_permeate_flow = 0.8 * Q_IN; % Desired permeate flow [L/h]

    % Initial bounds for membrane area A (m^2)
    A_min =0.1*10e-6;  % Minimum possible area
    A_max = 10;    % Arbitrary maximum area
    tolerance = 1e-6;  % Tolerance for convergence
    max_iter = 100;    % Maximum iterations for bisection method

    % Bisection method to find A
    for iter = 1:max_iter
        % Midpoint of current range for A
        A_mid = (A_min + A_max) / 2;

        % Calculate permeate flow using the updated equation
        permeate_flow = A_mid * Res * P; % [L/h]

        % Check convergence
        if abs(permeate_flow - desired_permeate_flow) < tolerance
            break;  % Converged to the solution
        elseif permeate_flow > desired_permeate_flow
            A_max = A_mid;  % Adjust upper bound
        else
            A_min = A_mid;  % Adjust lower bound
        end
    end

    % Output the membrane area
    y = A_mid;  % Membrane area (m^2)
end

== matlab function Final_openloop/MATLAB Function2 ==
  data: u input; y output
function y = Flow(u)
% Flow Function to calculate the required flow rate for a given concentration
% Inputs:
% u(1) - C1: Original concentration (g/L)
% u(2) - f1: Original flow rate (L/h)
% u(3) - C2: New concentration (g/L)
%
% Output:
% y - f2: Required flow rate (L/h) to achieve the same total mass flow T

% Input assignments
C1 = u(1);  % Original concentration (g/L)
f1 = u(2);  % Original flow rate (L/h)
C2 = u(3);  % New concentration (g/L)

% Calculate the required flow rate f2
y = (C1 * f1) / C2;  % New flow rate to maintain the same total mass flow

% Ensure the output is between 5 and 8
if y < 0.000001
    y = 0.000001;
elseif y > 8
    y = 8;
end

end

== matlab function Final_openloop/MATLAB Function7 ==
  data: u input; y output
function y = Flow(u)
% Flow Function to calculate the required flow rate for a given concentration
% Inputs:
% u(1) - C1: Original concentration (g/L)
% u(2) - f1: Original flow rate (L/h)
% u(3) - C2: New concentration (g/L)
%
% Output:
% y - f2: Required flow rate (L/h) to achieve the same total mass flow T

% Input assignments
C1 = u(1);  % Original concentration (g/L)
f1 = u(2);  % Original flow rate (L/h)
C2 = u(3);  % New concentration (g/L)

% Calculate the required flow rate f2
y = (C1 * f1) / C2;  % New flow rate to maintain the same total mass flow

% Ensure the output is between 5 and 8
if y < 0.000001
    y = 0.000001;
elseif y > 8
    y = 8;
end

end

== matlab function Final_openloop/UF-101 ==
  data: u input; y output
function y  = UF(u)

%Input
C_X_4=u(1);
C_GLU_4=u(2);
C_N_4=u(3);
Q_IN=u(4);
P=u(5);

%% parameters for nanofiltration 

P_0 = 0.49;              % referece pressure (kPa)
alpha_0=10.2*10^12;      % reference value
n=0.5;                   % 
A=0.014;                 % membrane area (m^2)
eta_perm=1.0*10^-8;      % Viscosity (kPa*s)
m_x_c=7.7*10^-3;         % (kg)
R_m =1.26*10^12;         % (1/m)

% Calculate alpha based on P_TM
alpha = alpha_0 * (P / P_0)^n;

% Calculate R_C
R_C = alpha * (m_x_c) / A;

dim=8;
y=zeros(dim,1);

%% Rejection coefficients for different species
Rej=[-0.0250*P^4-0.0236*P^3+0.0927*P^2+0.4960*P+0.1979; 0.01; 0.01];

%% Output calculation
    y(1)=((P/(eta_perm * (R_m + R_C)))*A)*1000*3600; % Permeate flow (L/m^2/h)

    y(2)=Q_IN-y(1);                                  % Retentate flow

%% Species balances for retentate stream (calculated based on inflow and rejection)
    y(3)=(Q_IN*C_X_4)/(y(2)+y(1)*(1-Rej(1)));        %Biomass species balance retentate stream
    y(4)=(Q_IN*C_GLU_4)/(y(2)+y(1)*(1-Rej(2)));      %Glucose species balance retentate stream
    y(5)=(Q_IN*C_N_4)/(y(2)+y(1)*(1-Rej(3)));        %Nitrogen species balance retentate stream
   
%% Species concentrations in permeate stream (calculated based on rejection)    
    y(6)=y(3)*(1-Rej(1));                            %Biomass concentration in permeate stream
    y(7)=y(4)*(1-Rej(2));                            %Glucose concentration in permeate stream
    y(8)=y(5)*(1-Rej(3));                            %Nitrogen concentration in permeate stream

end

== matlab function Final_openloop/MATLAB Function10 ==
  data: u input; y output
function y = Flow(u)
% Flow Function to calculate the required flow rate for a given concentration
% Inputs:
% u(1) - C1: Original concentration (g/L)
% u(2) - f1: Original flow rate (L/h)
% u(3) - C2: New concentration (g/L)
%
% Output:
% y - f2: Required flow rate (L/h) to achieve the same total mass flow T

% Input assignments
C1 = u(1);  % Original concentration (g/L)
f1 = u(2);  % Original flow rate (L/h)
C2 = u(3);  % New concentration (g/L)

% Calculate the required flow rate f2
y = (C1 * f1) / C2;  % New flow rate to maintain the same total mass flow

% Ensure the output is between 5 and 8
if y < 0.000001
    y = 0.000001;
elseif y > 8
    y = 8;
end

end

== matlab function Final_openloop/Q, Out L//h ==
  data: u input; y output
function y = Q_OUT(u)

% inputs
Q_M=u(1);
Q_R=u(2);


y=zeros(1,1);
y(1)=Q_M+Q_R;

== matlab function Final_openloop/VSP-101 ==
  data: u input size=2; y output size=2
function y  = Pump(u)

%input
Q_C=u(1);
n=u(2);

dim=2;

y=zeros(dim,1);

% output

y(1)=Q_C;
y(2)=((-0.085*Q_C^2 - 0.0000329*Q_C*n + 0.0000155555555555556*n^2)*(997*9.81))/10^5;


end

== matlab function Final_openloop/VSP-204 ==
  data: u input size=2; y output size=2
function y  = Pump(u)

%input
Q_C=u(1);
n=u(2);



y=zeros(2,1);

%output

y(1)=Q_C;
y(2)=((-0.085*Q_C^2 - 0.0000329*Q_C*n + 0.0000155555555555556*n^2)*(997*9.81))/10^5;


end

== matlab function Final_openloop/UF-201 ==
  data: u input; y output
function y  = UF(u)

%input
C_X_4=u(1);
C_DIS_4=u(2);
C_PLASMID_4=u(3);
C_DE_4=u(4);
C_ENDO_4=u(5);
C_ALKA_4=u(6);
C_CH3CO2K_4=u(7);
Q_IN=u(8);
P=u(9);
A=u(10);

%% parameters for nanofiltration 

P_0 = 0.49;                     % referece pressure (kPa)
alpha_0=10.2*10^12;             % reference.
n=0.5;                          % 
eta_perm=1.0*10^-8;             % Viscosity (kPa*s)
m_x_c=7.7*10^-3;                % (kg)
R_m =1.26*10^12;                % (1/m)

% Calculate alpha based on P_TM
alpha = alpha_0 * (P / P_0)^n;

% Calculate R_C
R_C = alpha * (m_x_c) / A;


dim=16;
y=zeros(dim,1);

%% Rejection coefficients for different species
Rej=[-0.0250*P^4-0.0236*P^3+0.0927*P^2+0.4960*P+0.1979; -0.0250*P^4-0.0236*P^3+0.0927*P^2+0.4960*P+0.1979; 0.01; 0.01; 0.01; 0.01; 0.01];


%% Output calculation

    y(1)=((P/(eta_perm * (R_m + R_C)))*A)*1000*3600;    % Permeate flow (L/m^2/h)

    y(2)=Q_IN-y(1);                                     % Retentate
    
 %% Species balances for retentate stream (calculated based on inflow and rejection)
    y(3)=(Q_IN*C_X_4)/(y(2)+y(1)*(1-Rej(1)));           % Biomass species balance--retentate stream
    y(4)=(Q_IN*C_DIS_4)/(y(2)+y(1)*(1-Rej(2)));         % Cell disrupts species balance--retentate stream
    y(5)=(Q_IN*C_PLASMID_4)/(y(2)+y(1)*(1-Rej(3)));     % Plasmid species balance--retentate stream
    y(6)=(Q_IN*C_DE_4)/(y(2)+y(1)*(1-Rej(4)));          % Denaturated plasmid species balance--retentate stream
    y(7)=(Q_IN*C_ENDO_4)/(y(2)+y(1)*(1-Rej(5)));        % Endotoxin species balance--retentate stream
    y(8)=(Q_IN*C_ALKA_4)/(y(2)+y(1)*(1-Rej(6)));        % Alkaline buffer species balance--retentate stream
    y(9)=(Q_IN*C_CH3CO2K_4)/(y(2)+y(1)*(1-Rej(7)));     % Neutralization buffer species balance--retentate stream
   
%% Species concentrations in permeate stream (calculated based on rejection)      
    y(10)=y(3)*(1-Rej(1));                              % Biomass concentration in permeate stream
    y(11)=y(4)*(1-Rej(2));                              % Cell disrupt concentration in permeate stream
    y(12)=y(5)*(1-Rej(3));                              % Plasmid concentration in permeate stream
    y(13)=y(6)*(1-Rej(4));                              % Denaturated plasmid concentration in permeate stream
    y(14)=y(7)*(1-Rej(5));                              % Endotoxin concentration in permeate stream
    y(15)=y(8)*(1-Rej(6));                              % Alkaline buffer concentration in permeate stream
    y(16)=y(9)*(1-Rej(7));                              % Neutralization buffer concentration in permeate stream
    

end

== matlab function Final_openloop/MATLAB Function4 ==
  data: u input; y output
function y = Resuspension (u)

% inputs
Q=u(1);
C_X_S=u(2);
C_NaOH=u(3);

%reaction
Q_resuspension=Q*10;
Q_Alkaline=Q_resuspension;


y=zeros(1,3);
y(1) = (C_X_S*Q)/(Q+Q_resuspension+Q_Alkaline);             %C_X_F
y(2) = (Q+Q_resuspension+Q_Alkaline);                       %Q total
y(3) = (C_NaOH*Q_Alkaline)/(Q+Q_resuspension+Q_Alkaline);   %NaOH
